simulink model "motor_clarke_park_model"  (R2023b)
settings: Solver=FixedStepDiscrete  StartTime=0.0  StopTime=0.001  FixedStep=0.001  RelTol=1e-3
settings Model: DataDictionary=motor_interface.sldd  Creator=user  LastModifiedBy=user
settings OptimizationCC: DefaultParameterBehavior=Inlined  EnhancedBackFolding=on  PassReuseOutputArgsAs=Individual arguments  OptimizeBlockOrder=speed  DifferentSizesBufferReuse=on  OptimizationCustomize=off  EfficientTunableParamExpr=on
settings DebuggingCC: ParameterTunabilityLossMsg=error
settings HardwareCC: ProdBitPerPointer=32  ProdBitPerSizeT=32  ProdBitPerPtrDiffT=32  ProdLargestAtomicInteger=Long  ProdLargestAtomicFloat=Double  ProdWordSize=32  ProdHWDeviceType=ARM Compatible->ARM Cortex  TargetLargestAtomicInteger=Long  TargetLargestAtomicFloat=Double  TargetIntDivRoundTo=Zero  TargetEndianess=LittleEndian  TargetHWDeviceType=ARM Compatible->ARM Cortex  ProdEqTarget=off
settings SFSimCC: MATLABDynamicMemAlloc=off
settings RTWCC: Description=Embedded Coder  SystemTargetFile=ert.tlc  GenCodeOnly=on  TemplateMakefile=ert_default_tmf  GenerateReport=on
settings CodeAppCC: ForceParamTrailComments=on  IgnoreCustomStorageClasses=off  OperatorAnnotations=on  SimulinkDataObjDesc=on  SFDataObjDesc=on  InsertBlockDesc=on
settings ERTTargetCC: TargetLangStandard=C99 (ISO)  CodeInterfacePackaging=Reusable function  InlinedParameterPlacement=NonHierarchical  ERTCustomFileTemplate=example_file_process.tlc

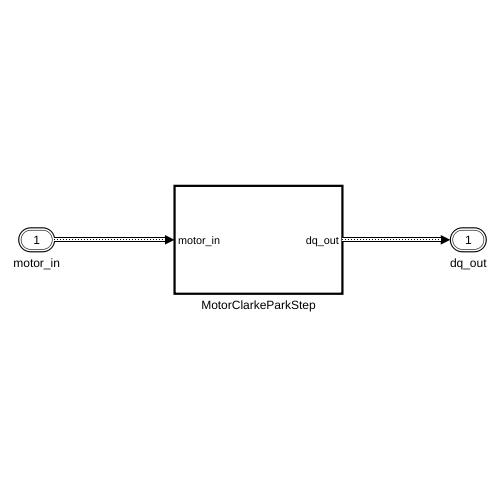
[thumbnail: Simulink's stored preview of the top-level diagram]
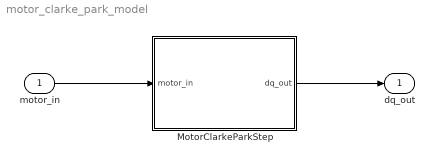
== system motor_clarke_park_model ==
  motor_in : Inport  OutDataTypeStr=Bus: motor_t  PortDimensions=1  BusOutputAsStruct=on
  MotorClarkeParkStep : Subsystem  TreatAsAtomicUnit=on  RTWFcnName=MotorClarkeParkStep  RTWFileName=MotorClarkeParkStep
      settings: RTWFcnNameOpts=User specified  RTWFileNameOpts=User specified
  dq_out : Outport  OutDataTypeStr=Bus: motor_dq_t  PortDimensions=1
  wires:
  motor_in/1 -> MotorClarkeParkStep/1(motor_in)
  MotorClarkeParkStep/1(dq_out) -> dq_out/1

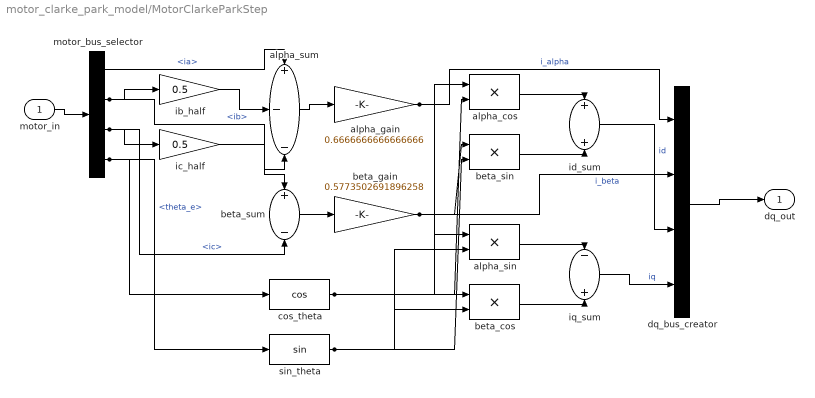
== system motor_clarke_park_model/MotorClarkeParkStep ==
  motor_in : Inport  OutDataTypeStr=Bus: motor_t  BusOutputAsStruct=on
  alpha_cos : Product  Inputs=**  OutDataTypeStr=T_MotorCurrent  SaturateOnIntegerOverflow=on
  alpha_gain : Gain  Gain=0.6666666666666666  ParamDataTypeStr=T_MotorCurrent  OutDataTypeStr=T_MotorCurrent  SaturateOnIntegerOverflow=on
  alpha_sin : Product  Inputs=**  OutDataTypeStr=T_MotorCurrent  SaturateOnIntegerOverflow=on
  alpha_sum : Sum  Inputs=+--  OutDataTypeStr=T_MotorCurrent  AccumDataTypeStr=T_MotorCurrent  SaturateOnIntegerOverflow=on
  beta_cos : Product  Inputs=**  OutDataTypeStr=T_MotorCurrent  SaturateOnIntegerOverflow=on
  beta_gain : Gain  Gain=0.5773502691896258  ParamDataTypeStr=T_MotorCurrent  OutDataTypeStr=T_MotorCurrent  SaturateOnIntegerOverflow=on
  beta_sin : Product  Inputs=**  OutDataTypeStr=T_MotorCurrent  SaturateOnIntegerOverflow=on
  beta_sum : Sum  Inputs=+-  OutDataTypeStr=T_MotorCurrent  AccumDataTypeStr=T_MotorCurrent  SaturateOnIntegerOverflow=on
  cos_theta : Trigonometry  Operator=cos
  dq_bus_creator : BusCreator  Inputs=4  OutDataTypeStr=Bus: motor_dq_t  NonVirtualBus=on
  ib_half : Gain  Gain=0.5  ParamDataTypeStr=T_MotorCurrent  OutDataTypeStr=T_MotorCurrent  SaturateOnIntegerOverflow=on
  ic_half : Gain  Gain=0.5  ParamDataTypeStr=T_MotorCurrent  OutDataTypeStr=T_MotorCurrent  SaturateOnIntegerOverflow=on
  id_sum : Sum  OutDataTypeStr=T_MotorCurrent  AccumDataTypeStr=T_MotorCurrent  SaturateOnIntegerOverflow=on
  iq_sum : Sum  Inputs=-+  OutDataTypeStr=T_MotorCurrent  AccumDataTypeStr=T_MotorCurrent  SaturateOnIntegerOverflow=on
  motor_bus_selector : BusSelector  OutputSignals=ia,ib,ic,theta_e
  sin_theta : Trigonometry
  dq_out : Outport  OutDataTypeStr=Bus: motor_dq_t
  wires:
  motor_in/1 -> motor_bus_selector/1
  motor_bus_selector/1 -> alpha_sum/1  "<ia>"
  motor_bus_selector/2 -> ib_half/1, beta_sum/1  "<ib>"
  motor_bus_selector/3 -> ic_half/1, beta_sum/2  "<ic>"
  ib_half/1 -> alpha_sum/2
  ic_half/1 -> alpha_sum/3
  alpha_sum/1 -> alpha_gain/1
  beta_sum/1 -> beta_gain/1
  motor_bus_selector/4 -> cos_theta/1, sin_theta/1  "<theta_e>"
  alpha_gain/1 -> alpha_cos/1, alpha_sin/1, dq_bus_creator/1  "i_alpha"
  cos_theta/1 -> alpha_cos/2, beta_cos/2
  beta_gain/1 -> beta_sin/1, beta_cos/1, dq_bus_creator/2  "i_beta"
  sin_theta/1 -> beta_sin/2, alpha_sin/2
  alpha_cos/1 -> id_sum/1
  beta_sin/1 -> id_sum/2
  alpha_sin/1 -> iq_sum/1
  beta_cos/1 -> iq_sum/2
  id_sum/1 -> dq_bus_creator/3  "id"
  iq_sum/1 -> dq_bus_creator/4  "iq"
  dq_bus_creator/1 -> dq_out/1
